simulink model "Test_DMP"  (R2018a)
settings: Solver=VariableStepAuto  StartTime=0.0  StopTime=2*tau  RelTol=1e-3
values from neighbouring files (symbols this model uses):
  Am = repmat(Am,1,6/length(Am))    [CostFCN.m]    (also in optimizeRobotMotion_openLoop.m; pFinal_runSim.m; simWalker_constraint.m)
  dt = .01    (= 0.01)    [Trajectory.m]    (also in rcp.m = 0.001)
  init_pos = Am'.*init_pos    [CostFCN.m]    (also in optimizeRobotMotion_openLoop.m; pFinal_runSim.m; simWalker_constraint.m)
  init_vel = Am'.*init_vel    [CostFCN.m]    (also in optimizeRobotMotion_openLoop.m; pFinal_runSim.m; simWalker_constraint.m)
  tau = params(1,2)    [CostFCN.m]    (also in Test_params.m = tau_nom; Trajectory.m = (2*pi)/omega; optimizeRobotMotion_openLoop.m = pFinal(1,2); pFinal_runSim.m = pFinal(1,2))
  Ym = Ym.*Am    [CostFCN.m]    (also in optimizeRobotMotion_openLoop.m; pFinal_runSim.m; simWalker_constraint.m)
undefined symbols (not defined in the file or in its folder): init_pos2, init_vel2, W, W2, Ym2
libraries: simulink_extras x6
(part 1 of 2)
settings Model: Creator=nozaripo  LastModifiedBy=nozaripo

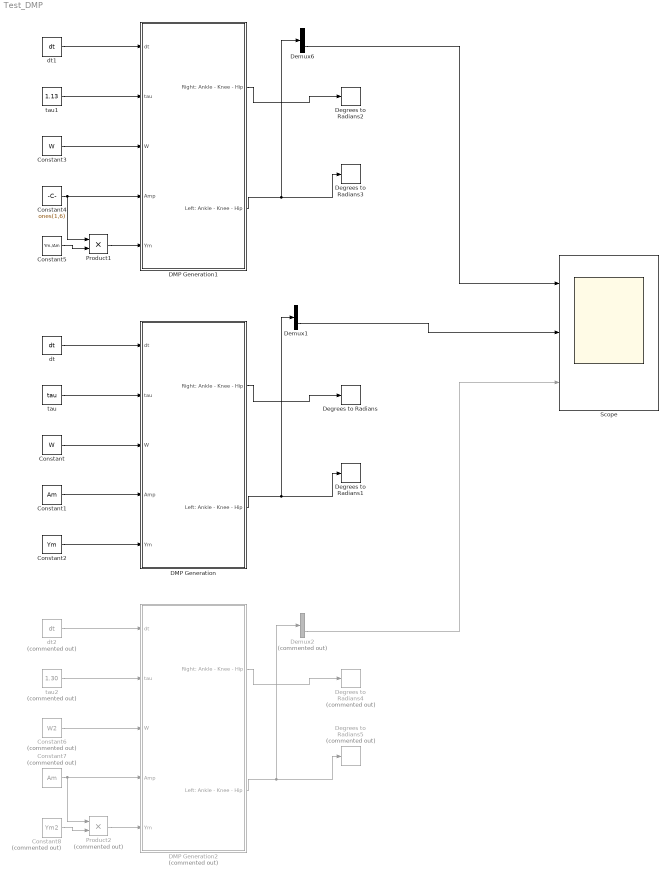
== system Test_DMP ==
  Constant : Constant  Value=W
  Constant1 : Constant  Value=Am
  Constant2 : Constant  Value=Ym
  Constant3 : Constant  Value=W
  Constant4 : Constant  Value=ones(1,6)
  Constant5 : Constant  Value=Ym./Am
  Constant6 : Constant  Commented=on  Value=W2
  Constant7 : Constant  Commented=on  Value=Am
  Constant8 : Constant  Commented=on  Value=Ym2
  DMP Generation : Subsystem
  DMP Generation1 : Subsystem
  DMP Generation2 : Subsystem  Commented=on
  Degrees to Radians{,1..3} (4 alike) : simulink_extras/Transformations/Degrees to Radians
  Degrees to Radians4 : simulink_extras/Transformations/Degrees to Radians  Commented=on
  Degrees to Radians5 : simulink_extras/Transformations/Degrees to Radians  Commented=on
  Demux1 : Demux  Outputs=3
  Demux2 : Demux  Commented=on  Outputs=3
  Demux6 : Demux  Outputs=3
  Product1 : Product
  Product2 : Product  Commented=on
  Scope : Scope  NumInputPorts=3
  dt : Constant  Value=dt
  dt1 : Constant  Value=dt
  dt2 : Constant  Commented=on  Value=dt
  tau : Constant  Value=tau
  tau1 : Constant  Value=1.13
  tau2 : Constant  Commented=on  Value=1.30
  wires:
  DMP Generation/2(Left: Ankle - Knee - Hip) -> Demux1/1, Degrees to Radians1/1
  DMP Generation/1(Right: Ankle - Knee - Hip) -> Degrees to Radians/1
  Constant/1 -> DMP Generation/3(W)
  Constant1/1 -> DMP Generation/4(Amp)
  Constant2/1 -> DMP Generation/5(Ym)
  tau/1 -> DMP Generation/2(tau)
  dt/1 -> DMP Generation/1(dt)
  dt1/1 -> DMP Generation1/1(dt)
  tau1/1 -> DMP Generation1/2(tau)
  Constant5/1 -> Product1/2
  Constant4/1 -> Product1/1, DMP Generation1/4(Amp)
  Constant3/1 -> DMP Generation1/3(W)
  DMP Generation1/1(Right: Ankle - Knee - Hip) -> Degrees to Radians2/1
  DMP Generation1/2(Left: Ankle - Knee - Hip) -> Demux6/1, Degrees to Radians3/1
  DMP Generation2/1(Right: Ankle - Knee - Hip) -> Degrees to Radians4/1
  DMP Generation2/2(Left: Ankle - Knee - Hip) -> Demux2/1, Degrees to Radians5/1
  Demux6/3 -> Scope/1
  Demux1/3 -> Scope/2
  Demux2/3 -> Scope/3
  Product1/1 -> DMP Generation1/5(Ym)
  Product2/1 -> DMP Generation2/5(Ym)
  Constant7/1 -> Product2/1, DMP Generation2/4(Amp)
  tau2/1 -> DMP Generation2/2(tau)
  Constant6/1 -> DMP Generation2/3(W)
  dt2/1 -> DMP Generation2/1(dt)
  Constant8/1 -> Product2/2

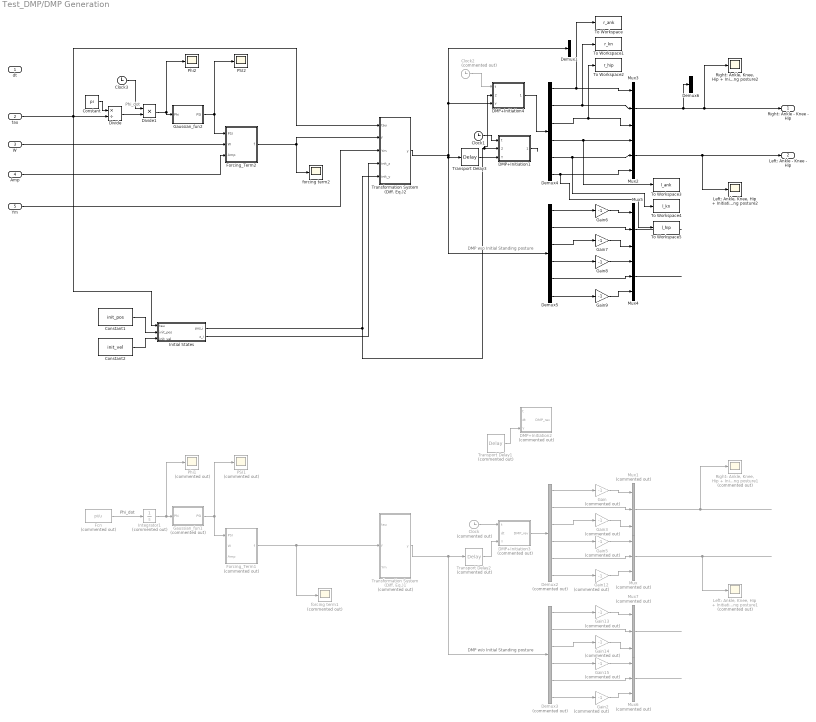
== system Test_DMP/DMP Generation ==
  note: Phi_dot
  note: DMP w/o Initial Standing posture
  note: Phi_dot
  note: DMP w/o Initial Standing posture
  dt : Inport
  tau : Inport  Port=2
  W : Inport  Port=3
  Amp : Inport  Port=4
  Ym : Inport  Port=5
  Clock : Clock  Commented=on
  Clock1 : Clock
  Clock2 : Clock  Commented=on
  Clock3 : Clock
  Constant : Constant  Value=pi
  Constant1 : Constant  Value=init_pos
  Constant2 : Constant  Value=init_vel
  DMP+Initiation1 : MATLAB Function  TreatAsAtomicUnit=on
  DMP+Initiation2 : MATLAB Function  Commented=on  TreatAsAtomicUnit=on
  DMP+Initiation3 : MATLAB Function  Commented=on  TreatAsAtomicUnit=on
  DMP+Initiation4 : MATLAB Function  TreatAsAtomicUnit=on
  Demux1 : Demux  Outputs=2
  Demux2 : Demux  Commented=on  Outputs=6
  Demux3 : Demux  Commented=on  Outputs=6
  Demux4 : Demux  Outputs=6
  Demux5 : Demux  Outputs=6
  Demux6 : Demux  Outputs=3
  Divide : Product  Inputs=*/
  Divide1 : Product  Inputs=**
  Fcn : Fcn  Commented=on  Expr=pi/u
  Forcing_Term1 : MATLAB Function  Commented=on  TreatAsAtomicUnit=on
  Forcing_Term2 : MATLAB Function  TreatAsAtomicUnit=on
  Gain{,2..3,5,12..15} (8 alike) : Gain  Commented=on  Gain=-1
  Gain{6..9} (4 alike) : Gain  Gain=-1
  Gaussian_fun1 : MATLAB Function  Commented=on  TreatAsAtomicUnit=on
  Gaussian_fun2 : MATLAB Function  TreatAsAtomicUnit=on
  Initial States : MATLAB Function  TreatAsAtomicUnit=on
  Integrator1 : Integrator  Commented=on
  "Left: Ankle, Knee, Hip + Initiatial standing posture1" : Scope  Commented=on
  "Left: Ankle, Knee, Hip + Initiatial standing posture2" : Scope
  Mux{,1,6..7} (4 alike) : Mux  Commented=on  Inputs=3
  Mux{2..5} (4 alike) : Mux  Inputs=3
  PSI1 : Scope  Commented=on
  PSI2 : Scope
  Phi1 : Scope  Commented=on
  Phi2 : Scope
  "Right: Ankle, Knee, Hip + Initiatial standing posture1" : Scope  Commented=on
  "Right: Ankle, Knee, Hip + Initiatial standing posture2" : Scope
  To Workspace : ToWorkspace  VariableName=r_ank  SampleTime=-1
      settings: Save2DSignal=2-D array (concatenate along first dimension)
  To Workspace1 : ToWorkspace  VariableName=r_kn  SampleTime=-1
      settings: Save2DSignal=2-D array (concatenate along first dimension)
  To Workspace2 : ToWorkspace  VariableName=r_hip  SampleTime=-1
      settings: Save2DSignal=2-D array (concatenate along first dimension)
  To Workspace3 : ToWorkspace  VariableName=l_ank  SampleTime=-1
      settings: Save2DSignal=2-D array (concatenate along first dimension)
  To Workspace4 : ToWorkspace  VariableName=l_kn  SampleTime=-1
      settings: Save2DSignal=2-D array (concatenate along first dimension)
  To Workspace5 : ToWorkspace  VariableName=l_hip  SampleTime=-1
      settings: Save2DSignal=2-D array (concatenate along first dimension)
  Transformation System (Diff. Eq.)1 : Subsystem  Commented=on
  Transformation System (Diff. Eq.)2 : Subsystem
  Transport Delay1 : TransportDelay  Commented=on  DelayTime=.45
  Transport Delay2 : TransportDelay  Commented=on  DelayTime=.55
  Transport Delay3 : TransportDelay  DelayTime=.67
  forcing term1 : Scope  Commented=on
  forcing term2 : Scope
  Right: Ankle - Knee - Hip : Outport
  Left: Ankle - Knee - Hip : Outport  Port=2
  wires:
  Demux2/3 -> Gain3/1
  Gain14/1 -> Mux7/3
  Demux2/5 -> Mux/2
  Demux2/6 -> Gain12/1
  Mux1/1 -> "Right: Ankle, Knee, Hip + Initiatial standing posture1"/1
  Demux3/5 -> Mux6/2
  Demux3/2 -> Mux7/2
  Gain3/1 -> Mux1/3
  Gain15/1 -> Mux6/1
  Demux2/4 -> Gain5/1
  Demux3/3 -> Gain14/1
  Mux6/1 -> ?
  Gaussian_fun1/1(PSI) -> PSI1/1, Forcing_Term1/1(PSI)
  Mux7/1 -> ?
  DMP+Initiation3/1(DMP_rev) -> Demux2/1
  Gain2/1 -> Mux6/3
  Transformation System (Diff. Eq.)1/1(y) -> Transport Delay2/1, Demux3/1
  Forcing_Term1/1(f) -> forcing term1/1, Transformation System (Diff. Eq.)1/2(f)
  Gain/1 -> Mux1/1
  Demux3/4 -> Gain15/1
  Mux/1 -> "Left: Ankle, Knee, Hip + Initiatial standing posture1"/1
  Fcn/1 -> Integrator1/1
  Demux2/2 -> Mux1/2
  Integrator1/1 -> Phi1/1, Gaussian_fun1/1(Phi)
  Gain5/1 -> Mux/1
  Demux3/1 -> Gain13/1
  Demux3/6 -> Gain2/1
  Demux2/1 -> Gain/1
  ? -> Forcing_Term1/3(Amp)
  ? -> Transformation System (Diff. Eq.)1/3(Ym)
  Gain12/1 -> Mux/3
  ? -> Fcn/1, Transformation System (Diff. Eq.)1/1(tau)
  ? -> Forcing_Term1/2(W)
  Gain13/1 -> Mux7/1
  ? -> DMP+Initiation2/1(t)
  Transport Delay1/1 -> DMP+Initiation2/3(Y)
  ? -> DMP+Initiation3/2(dt)
  Clock/1 -> DMP+Initiation3/1(t)
  Transport Delay2/1 -> DMP+Initiation3/3(Y)
  DMP+Initiation1/1(DMP_rev) -> ?
  Divide/1 -> Divide1/2
  Mux5/1 -> ?
  Forcing_Term2/1(f) -> Transformation System (Diff. Eq.)2/2(f), forcing term2/1
  Demux4/6 -> Mux2/3, To Workspace5/1
  Ym/1 -> Transformation System (Diff. Eq.)2/3(Ym)
  Demux5/1 -> Gain6/1
  Demux5/2 -> Mux5/2
  Mux2/1 -> Left: Ankle - Knee - Hip/1, "Left: Ankle, Knee, Hip + Initiatial standing posture2"/1
  Demux5/4 -> Gain8/1
  Transport Delay3/1 -> DMP+Initiation1/3(Y)
  Constant/1 -> Divide/1
  Demux4/5 -> To Workspace4/1, Mux2/2
  Gain9/1 -> Mux4/3
  Clock1/1 -> DMP+Initiation1/1(t)
  Gain8/1 -> Mux4/1
  Demux4/3 -> Mux3/3, To Workspace2/1
  Gain7/1 -> Mux5/3
  Demux5/3 -> Gain7/1
  Demux5/6 -> Gain9/1
  Amp/1 -> Forcing_Term2/3(Amp)
  Demux5/5 -> Mux4/2
  Gaussian_fun2/1(PSI) -> PSI2/1, Forcing_Term2/1(PSI)
  W/1 -> Forcing_Term2/2(W)
  Demux4/4 -> Mux2/1, To Workspace3/1
  Demux4/1 -> Mux3/1, To Workspace/1
  Mux4/1 -> ?
  Transformation System (Diff. Eq.)2/1(y) -> Transport Delay3/1, Demux5/1, DMP+Initiation4/3(Y), Demux1/1
  Demux4/2 -> To Workspace1/1, Mux3/2
  Mux3/1 -> Demux6/1, Right: Ankle - Knee - Hip/1, "Right: Ankle, Knee, Hip + Initiatial standing posture2"/1
  Divide1/1 -> Gaussian_fun2/1(Phi), Phi2/1
  Gain6/1 -> Mux5/1
  Constant2/1 -> Initial States/3(init_vel)
  Constant1/1 -> Initial States/2(init_pos)
  Initial States/2(z_i) -> Transformation System (Diff. Eq.)2/4(init_z)
  Initial States/1(pos_i) -> Transformation System (Diff. Eq.)2/5(init_y), DMP+Initiation4/2(init_pos), DMP+Initiation1/2(init_pos)
  tau/1 -> Transformation System (Diff. Eq.)2/1(tau), Initial States/1(tau), Divide/2
  Clock2/1 -> DMP+Initiation4/1(t)
  DMP+Initiation4/1(DMP_rev) -> Demux4/1
  Clock3/1 -> Divide1/1

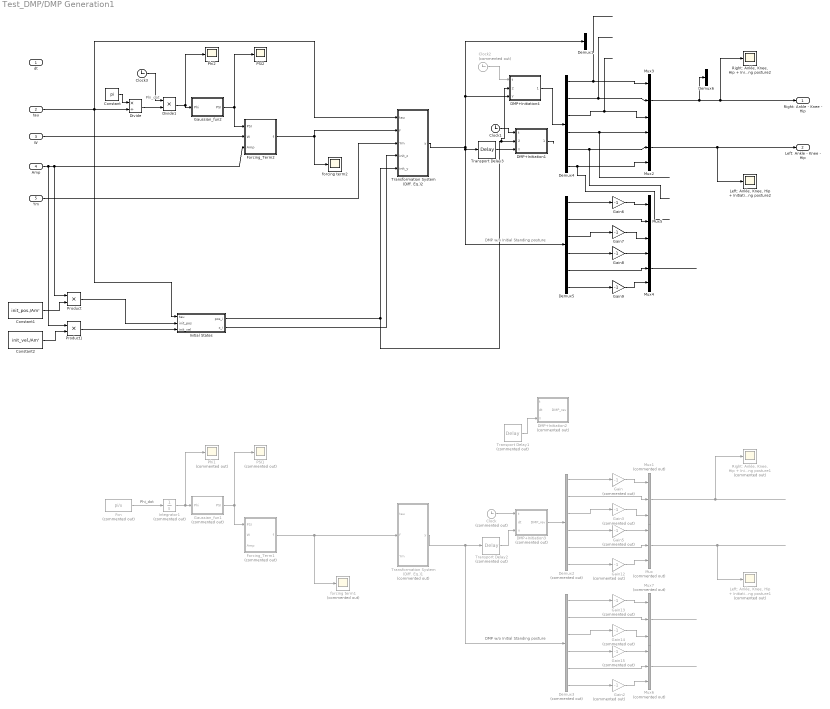
== system Test_DMP/DMP Generation1 ==
  note: DMP w/o Initial Standing posture
  note: Phi_dot
  note: DMP w/o Initial Standing posture
  note: Phi_dot
  dt : Inport
  tau : Inport  Port=2
  W : Inport  Port=3
  Amp : Inport  Port=4
  Ym : Inport  Port=5
  Clock : Clock  Commented=on
  Clock1 : Clock
  Clock2 : Clock  Commented=on
  Clock3 : Clock
  Constant : Constant  Value=pi
  Constant1 : Constant  Value=init_pos./Am'
  Constant2 : Constant  Value=init_vel./Am'
  DMP+Initiation1 : MATLAB Function  TreatAsAtomicUnit=on
  DMP+Initiation2 : MATLAB Function  Commented=on  TreatAsAtomicUnit=on
  DMP+Initiation3 : MATLAB Function  Commented=on  TreatAsAtomicUnit=on
  DMP+Initiation4 : MATLAB Function  TreatAsAtomicUnit=on
  Demux1 : Demux  Outputs=2
  Demux2 : Demux  Commented=on  Outputs=6
  Demux3 : Demux  Commented=on  Outputs=6
  Demux4 : Demux  Outputs=6
  Demux5 : Demux  Outputs=6
  Demux6 : Demux  Outputs=3
  Divide : Product  Inputs=*/
  Divide1 : Product  Inputs=**
  Fcn : Fcn  Commented=on  Expr=pi/u
  Forcing_Term1 : MATLAB Function  Commented=on  TreatAsAtomicUnit=on
  Forcing_Term2 : MATLAB Function  TreatAsAtomicUnit=on
  Gain{,2..3,5,12..15} (8 alike) : Gain  Commented=on  Gain=-1
  Gain{6..9} (4 alike) : Gain  Gain=-1
  Gaussian_fun1 : MATLAB Function  Commented=on  TreatAsAtomicUnit=on
  Gaussian_fun2 : MATLAB Function  TreatAsAtomicUnit=on
  Initial States : MATLAB Function  TreatAsAtomicUnit=on
  Integrator1 : Integrator  Commented=on
  "Left: Ankle, Knee, Hip + Initiatial standing posture1" : Scope  Commented=on
  "Left: Ankle, Knee, Hip + Initiatial standing posture2" : Scope
  Mux{,1,6..7} (4 alike) : Mux  Commented=on  Inputs=3
  Mux{2..5} (4 alike) : Mux  Inputs=3
  PSI1 : Scope  Commented=on
  PSI2 : Scope
  Phi1 : Scope  Commented=on
  Phi2 : Scope
  Product : Product
  Product1 : Product
  "Right: Ankle, Knee, Hip + Initiatial standing posture1" : Scope  Commented=on
  "Right: Ankle, Knee, Hip + Initiatial standing posture2" : Scope
  Transformation System (Diff. Eq.)1 : Subsystem  Commented=on
  Transformation System (Diff. Eq.)2 : Subsystem
  Transport Delay1 : TransportDelay  Commented=on  DelayTime=.45
  Transport Delay2 : TransportDelay  Commented=on  DelayTime=.55
  Transport Delay3 : TransportDelay  DelayTime=.67
  forcing term1 : Scope  Commented=on
  forcing term2 : Scope
  Right: Ankle - Knee - Hip : Outport
  Left: Ankle - Knee - Hip : Outport  Port=2
  wires:
  Clock3/1 -> Divide1/1
  DMP+Initiation4/1(DMP_rev) -> Demux4/1
  Clock2/1 -> DMP+Initiation4/1(t)
  tau/1 -> Divide/2, Initial States/1(tau), Transformation System (Diff. Eq.)2/1(tau)
  Initial States/1(pos_i) -> DMP+Initiation1/2(init_pos), DMP+Initiation4/2(init_pos), Transformation System (Diff. Eq.)2/5(init_y)
  Initial States/2(z_i) -> Transformation System (Diff. Eq.)2/4(init_z)
  Constant1/1 -> Product/2
  Gain6/1 -> Mux5/1
  Divide1/1 -> Phi2/1, Gaussian_fun2/1(Phi)
  Mux3/1 -> "Right: Ankle, Knee, Hip + Initiatial standing posture2"/1, Right: Ankle - Knee - Hip/1, Demux6/1
  Demux4/2 -> Mux3/2
  Transformation System (Diff. Eq.)2/1(y) -> Demux1/1, DMP+Initiation4/3(Y), Demux5/1, Transport Delay3/1
  Mux4/1 -> ?
  Demux4/1 -> Mux3/1
  Demux4/4 -> Mux2/1
  W/1 -> Forcing_Term2/2(W)
  Gaussian_fun2/1(PSI) -> Forcing_Term2/1(PSI), PSI2/1
  Demux5/5 -> Mux4/2
  Amp/1 -> Product1/1, Product/1, Forcing_Term2/3(Amp)
  Demux5/6 -> Gain9/1
  Demux5/3 -> Gain7/1
  Gain7/1 -> Mux5/3
  Demux4/3 -> Mux3/3
  Gain8/1 -> Mux4/1
  Clock1/1 -> DMP+Initiation1/1(t)
  Gain9/1 -> Mux4/3
  Demux4/5 -> Mux2/2
  Constant/1 -> Divide/1
  Transport Delay3/1 -> DMP+Initiation1/3(Y)
  Demux5/4 -> Gain8/1
  Mux2/1 -> "Left: Ankle, Knee, Hip + Initiatial standing posture2"/1, Left: Ankle - Knee - Hip/1
  Demux5/2 -> Mux5/2
  Demux5/1 -> Gain6/1
  Ym/1 -> Transformation System (Diff. Eq.)2/3(Ym)
  Demux4/6 -> Mux2/3
  Forcing_Term2/1(f) -> forcing term2/1, Transformation System (Diff. Eq.)2/2(f)
  Divide/1 -> Divide1/2
  DMP+Initiation1/1(DMP_rev) -> ?
  Transport Delay2/1 -> DMP+Initiation3/3(Y)
  Clock/1 -> DMP+Initiation3/1(t)
  ? -> DMP+Initiation3/2(dt)
  Transport Delay1/1 -> DMP+Initiation2/3(Y)
  ? -> DMP+Initiation2/1(t)
  Gain13/1 -> Mux7/1
  ? -> Forcing_Term1/2(W)
  ? -> Transformation System (Diff. Eq.)1/1(tau), Fcn/1
  Gain12/1 -> Mux/3
  ? -> Transformation System (Diff. Eq.)1/3(Ym)
  ? -> Forcing_Term1/3(Amp)
  Demux2/1 -> Gain/1
  Demux3/6 -> Gain2/1
  Demux3/1 -> Gain13/1
  Gain5/1 -> Mux/1
  Integrator1/1 -> Gaussian_fun1/1(Phi), Phi1/1
  Demux2/2 -> Mux1/2
  Fcn/1 -> Integrator1/1
  Mux/1 -> "Left: Ankle, Knee, Hip + Initiatial standing posture1"/1
  Demux3/4 -> Gain15/1
  Gain/1 -> Mux1/1
  Forcing_Term1/1(f) -> Transformation System (Diff. Eq.)1/2(f), forcing term1/1
  Transformation System (Diff. Eq.)1/1(y) -> Demux3/1, Transport Delay2/1
  Gain2/1 -> Mux6/3
  DMP+Initiation3/1(DMP_rev) -> Demux2/1
  Mux7/1 -> ?
  Gaussian_fun1/1(PSI) -> Forcing_Term1/1(PSI), PSI1/1
  Mux6/1 -> ?
  Demux3/3 -> Gain14/1
  Demux2/4 -> Gain5/1
  Gain15/1 -> Mux6/1
  Gain3/1 -> Mux1/3
  Demux3/2 -> Mux7/2
  Demux3/5 -> Mux6/2
  Mux1/1 -> "Right: Ankle, Knee, Hip + Initiatial standing posture1"/1
  Demux2/6 -> Gain12/1
  Demux2/5 -> Mux/2
  Gain14/1 -> Mux7/3
  Demux2/3 -> Gain3/1
  Product/1 -> Initial States/2(init_pos)
  Constant2/1 -> Product1/2
  Product1/1 -> Initial States/3(init_vel)

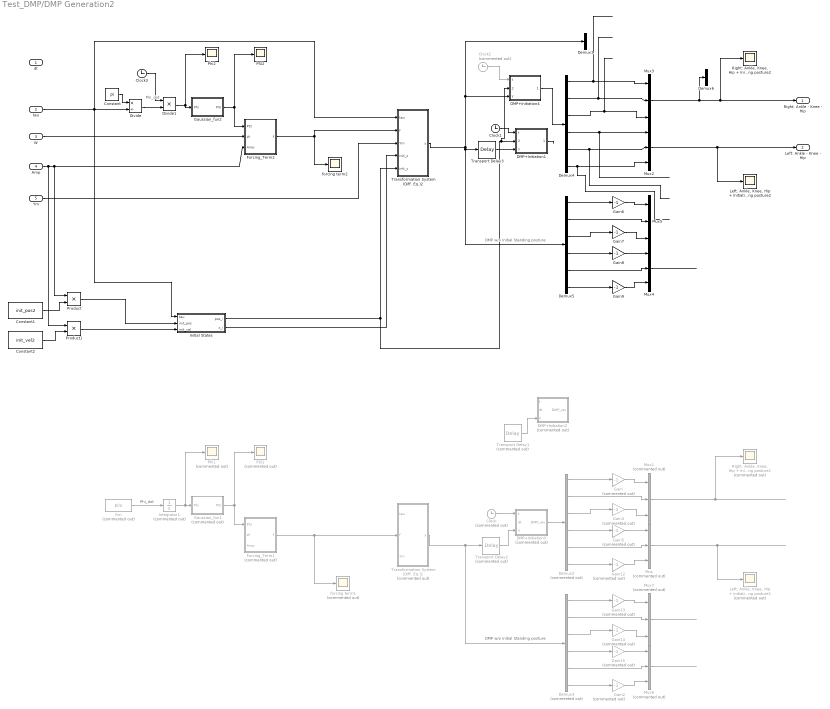
== system Test_DMP/DMP Generation2 ==
  note: DMP w/o Initial Standing posture
  note: Phi_dot
  note: DMP w/o Initial Standing posture
  note: Phi_dot
  dt : Inport
  tau : Inport  Port=2
  W : Inport  Port=3
  Amp : Inport  Port=4
  Ym : Inport  Port=5
  Clock : Clock  Commented=on
  Clock1 : Clock
  Clock2 : Clock  Commented=on
  Clock3 : Clock
  Constant : Constant  Value=pi
  Constant1 : Constant  Value=init_pos2
  Constant2 : Constant  Value=init_vel2
  DMP+Initiation1 : MATLAB Function  TreatAsAtomicUnit=on
  DMP+Initiation2 : MATLAB Function  Commented=on  TreatAsAtomicUnit=on
  DMP+Initiation3 : MATLAB Function  Commented=on  TreatAsAtomicUnit=on
  DMP+Initiation4 : MATLAB Function  TreatAsAtomicUnit=on
  Demux1 : Demux  Outputs=2
  Demux2 : Demux  Commented=on  Outputs=6
  Demux3 : Demux  Commented=on  Outputs=6
  Demux4 : Demux  Outputs=6
  Demux5 : Demux  Outputs=6
  Demux6 : Demux  Outputs=3
  Divide : Product  Inputs=*/
  Divide1 : Product  Inputs=**
  Fcn : Fcn  Commented=on  Expr=pi/u
  Forcing_Term1 : MATLAB Function  Commented=on  TreatAsAtomicUnit=on
  Forcing_Term2 : MATLAB Function  TreatAsAtomicUnit=on
  Gain{,2..3,5,12..15} (8 alike) : Gain  Commented=on  Gain=-1
  Gain{6..9} (4 alike) : Gain  Gain=-1
  Gaussian_fun1 : MATLAB Function  Commented=on  TreatAsAtomicUnit=on
  Gaussian_fun2 : MATLAB Function  TreatAsAtomicUnit=on
  Initial States : MATLAB Function  TreatAsAtomicUnit=on
  Integrator1 : Integrator  Commented=on
  "Left: Ankle, Knee, Hip + Initiatial standing posture1" : Scope  Commented=on
  "Left: Ankle, Knee, Hip + Initiatial standing posture2" : Scope
  Mux{,1,6..7} (4 alike) : Mux  Commented=on  Inputs=3
  Mux{2..5} (4 alike) : Mux  Inputs=3
  PSI1 : Scope  Commented=on
  PSI2 : Scope
  Phi1 : Scope  Commented=on
  Phi2 : Scope
  Product : Product
  Product1 : Product
  "Right: Ankle, Knee, Hip + Initiatial standing posture1" : Scope  Commented=on
  "Right: Ankle, Knee, Hip + Initiatial standing posture2" : Scope
  Transformation System (Diff. Eq.)1 : Subsystem  Commented=on
  Transformation System (Diff. Eq.)2 : Subsystem
  Transport Delay1 : TransportDelay  Commented=on  DelayTime=.45
  Transport Delay2 : TransportDelay  Commented=on  DelayTime=.55
  Transport Delay3 : TransportDelay  DelayTime=.67
  forcing term1 : Scope  Commented=on
  forcing term2 : Scope
  Right: Ankle - Knee - Hip : Outport
  Left: Ankle - Knee - Hip : Outport  Port=2
  wires:
  Clock3/1 -> Divide1/1
  DMP+Initiation4/1(DMP_rev) -> Demux4/1
  Clock2/1 -> DMP+Initiation4/1(t)
  tau/1 -> Divide/2, Initial States/1(tau), Transformation System (Diff. Eq.)2/1(tau)
  Initial States/1(pos_i) -> DMP+Initiation1/2(init_pos), DMP+Initiation4/2(init_pos), Transformation System (Diff. Eq.)2/5(init_y)
  Initial States/2(z_i) -> Transformation System (Diff. Eq.)2/4(init_z)
  Constant1/1 -> Product/2
  Gain6/1 -> Mux5/1
  Divide1/1 -> Phi2/1, Gaussian_fun2/1(Phi)
  Mux3/1 -> "Right: Ankle, Knee, Hip + Initiatial standing posture2"/1, Right: Ankle - Knee - Hip/1, Demux6/1
  Demux4/2 -> Mux3/2
  Transformation System (Diff. Eq.)2/1(y) -> Demux1/1, DMP+Initiation4/3(Y), Demux5/1, Transport Delay3/1
  Mux4/1 -> ?
  Demux4/1 -> Mux3/1
  Demux4/4 -> Mux2/1
  W/1 -> Forcing_Term2/2(W)
  Gaussian_fun2/1(PSI) -> Forcing_Term2/1(PSI), PSI2/1
  Demux5/5 -> Mux4/2
  Amp/1 -> Product1/1, Product/1, Forcing_Term2/3(Amp)
  Demux5/6 -> Gain9/1
  Demux5/3 -> Gain7/1
  Gain7/1 -> Mux5/3
  Demux4/3 -> Mux3/3
  Gain8/1 -> Mux4/1
  Clock1/1 -> DMP+Initiation1/1(t)
  Gain9/1 -> Mux4/3
  Demux4/5 -> Mux2/2
  Constant/1 -> Divide/1
  Transport Delay3/1 -> DMP+Initiation1/3(Y)
  Demux5/4 -> Gain8/1
  Mux2/1 -> "Left: Ankle, Knee, Hip + Initiatial standing posture2"/1, Left: Ankle - Knee - Hip/1
  Demux5/2 -> Mux5/2
  Demux5/1 -> Gain6/1
  Ym/1 -> Transformation System (Diff. Eq.)2/3(Ym)
  Demux4/6 -> Mux2/3
  Forcing_Term2/1(f) -> forcing term2/1, Transformation System (Diff. Eq.)2/2(f)
  Divide/1 -> Divide1/2
  DMP+Initiation1/1(DMP_rev) -> ?
  Transport Delay2/1 -> DMP+Initiation3/3(Y)
  Clock/1 -> DMP+Initiation3/1(t)
  ? -> DMP+Initiation3/2(dt)
  Transport Delay1/1 -> DMP+Initiation2/3(Y)
  ? -> DMP+Initiation2/1(t)
  Gain13/1 -> Mux7/1
  ? -> Forcing_Term1/2(W)
  ? -> Transformation System (Diff. Eq.)1/1(tau), Fcn/1
  Gain12/1 -> Mux/3
  ? -> Transformation System (Diff. Eq.)1/3(Ym)
  ? -> Forcing_Term1/3(Amp)
  Demux2/1 -> Gain/1
  Demux3/6 -> Gain2/1
  Demux3/1 -> Gain13/1
  Gain5/1 -> Mux/1
  Integrator1/1 -> Gaussian_fun1/1(Phi), Phi1/1
  Demux2/2 -> Mux1/2
  Fcn/1 -> Integrator1/1
  Mux/1 -> "Left: Ankle, Knee, Hip + Initiatial standing posture1"/1
  Demux3/4 -> Gain15/1
  Gain/1 -> Mux1/1
  Forcing_Term1/1(f) -> Transformation System (Diff. Eq.)1/2(f), forcing term1/1
  Transformation System (Diff. Eq.)1/1(y) -> Demux3/1, Transport Delay2/1
  Gain2/1 -> Mux6/3
  DMP+Initiation3/1(DMP_rev) -> Demux2/1
  Mux7/1 -> ?
  Gaussian_fun1/1(PSI) -> Forcing_Term1/1(PSI), PSI1/1
  Mux6/1 -> ?
  Demux3/3 -> Gain14/1
  Demux2/4 -> Gain5/1
  Gain15/1 -> Mux6/1
  Gain3/1 -> Mux1/3
  Demux3/2 -> Mux7/2
  Demux3/5 -> Mux6/2
  Mux1/1 -> "Right: Ankle, Knee, Hip + Initiatial standing posture1"/1
  Demux2/6 -> Gain12/1
  Demux2/5 -> Mux/2
  Gain14/1 -> Mux7/3
  Demux2/3 -> Gain3/1
  Product/1 -> Initial States/2(init_pos)
  Constant2/1 -> Product1/2
  Product1/1 -> Initial States/3(init_vel)

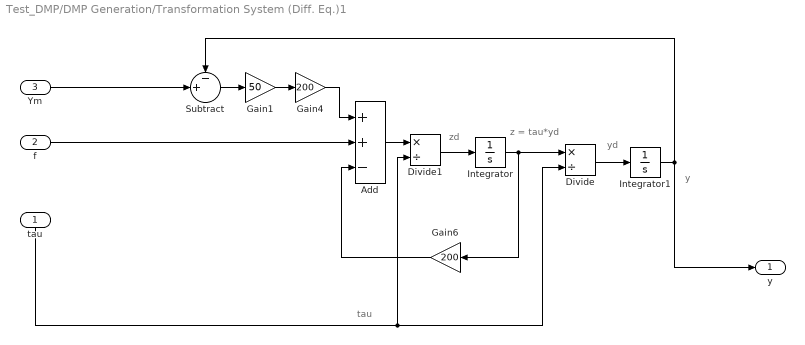
== system Test_DMP/DMP Generation/Transformation System (Diff. Eq.)1 ==
  note: y
  note: zd
  note: tau
  note: yd
  note: z = tau*yd
  tau : Inport
  f : Inport  Port=2
  Ym : Inport  Port=3
  Add : Sum  Inputs=++-
  Divide : Product  Inputs=*/
  Divide1 : Product  Inputs=*/
  Gain1 : Gain  Gain=50
  Gain4 : Gain  Gain=200
  Gain6 : Gain  Gain=200
  Integrator : Integrator
  Integrator1 : Integrator
  Subtract : Sum  Inputs=-+|
  y : Outport
  wires:
  Divide/1 -> Integrator1/1
  Add/1 -> Divide1/1
  Gain1/1 -> Gain4/1
  Gain4/1 -> Add/1
  Subtract/1 -> Gain1/1
  Divide1/1 -> Integrator/1
  tau/1 -> Divide/2, Divide1/2
  f/1 -> Add/2
  Integrator1/1 -> y/1, Subtract/1
  Integrator/1 -> Gain6/1, Divide/1
  Gain6/1 -> Add/3
  Ym/1 -> Subtract/2

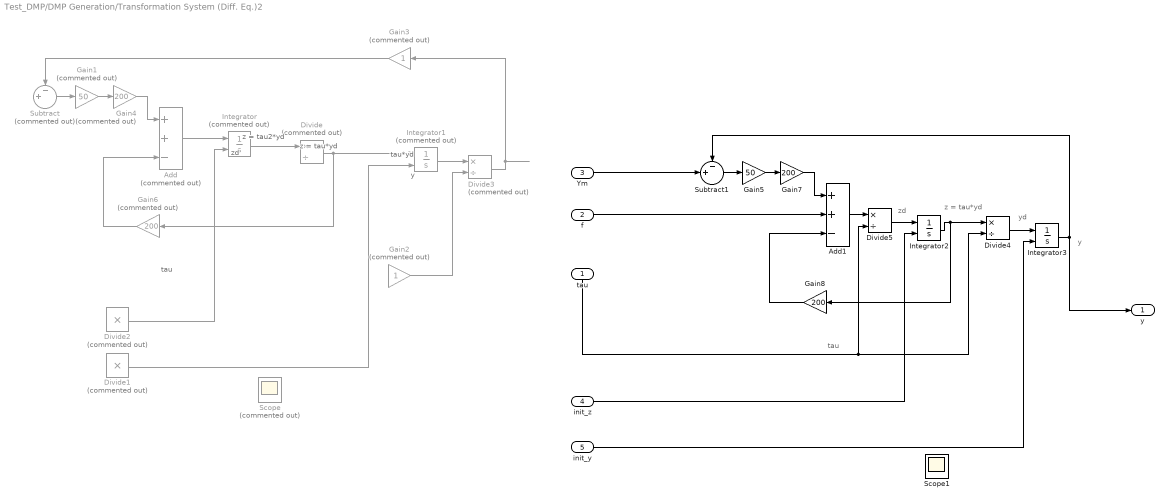
== system Test_DMP/DMP Generation/Transformation System (Diff. Eq.)2 ==
  note: y
  note: zd
  note: tau
  note: tau*yd
  note: z = tau2*yd
  note: z = tau*yd
  note: y
  note: zd
  note: tau
  note: yd
  note: z = tau*yd
  tau : Inport
  f : Inport  Port=2
  Ym : Inport  Port=3
  init_z : Inport  Port=4
  init_y : Inport  Port=5
  Add : Sum  Commented=on  Inputs=++-
  Add1 : Sum  Inputs=++-
  Divide : Product  Commented=on  Inputs=*/
  Divide1 : Product  Commented=on  Inputs=**
  Divide2 : Product  Commented=on  Inputs=**
  Divide3 : Product  Commented=on  Inputs=*/
  Divide4 : Product  Inputs=*/
  Divide5 : Product  Inputs=*/
  Gain1 : Gain  Commented=on  Gain=50
  Gain2 : Gain  Commented=on
  Gain3 : Gain  Commented=on
  Gain4 : Gain  Commented=on  Gain=200
  Gain5 : Gain  Gain=50
  Gain6 : Gain  Commented=on  Gain=200
  Gain7 : Gain  Gain=200
  Gain8 : Gain  Gain=200
  Integrator : Integrator  Commented=on  InitialConditionSource=external  LimitOutput=on
  Integrator1 : Integrator  Commented=on  InitialConditionSource=external
  Integrator2 : Integrator  InitialConditionSource=external
  Integrator3 : Integrator  InitialConditionSource=external
  Scope : Scope  Commented=on
  Scope1 : Scope
  Subtract : Sum  Commented=on  Inputs=-+|
  Subtract1 : Sum  Inputs=-+|
  y : Outport
  wires:
  Divide/1 -> Gain6/1, Integrator1/1
  Gain1/1 -> Gain4/1
  Gain4/1 -> Add/1
  Subtract/1 -> Gain1/1
  Add/1 -> Integrator/1
  ? -> Divide1/1, Divide2/1, Gain2/1, Divide/2
  ? -> Add/2
  Divide3/1 -> Gain3/1
  Integrator/1 -> Divide/1
  Gain6/1 -> Add/3
  ? -> Subtract/2
  ? -> Divide2/2
  ? -> Divide1/2
  Divide2/1 -> Integrator/2
  Divide1/1 -> Integrator1/2
  Integrator1/1 -> Divide3/1
  Gain2/1 -> Divide3/2
  Gain3/1 -> Subtract/1
  init_y/1 -> Integrator3/2
  Ym/1 -> Subtract1/2
  Integrator2/1 -> Gain8/1, Divide4/1
  init_z/1 -> Integrator2/2
  Gain8/1 -> Add1/3
  Integrator3/1 -> Subtract1/1, y/1
  f/1 -> Add1/2
  Divide5/1 -> Integrator2/1
  Gain7/1 -> Add1/1
  tau/1 -> Divide4/2, Divide5/2
  Subtract1/1 -> Gain5/1
  Gain5/1 -> Gain7/1
  Add1/1 -> Divide5/1
  Divide4/1 -> Integrator3/1

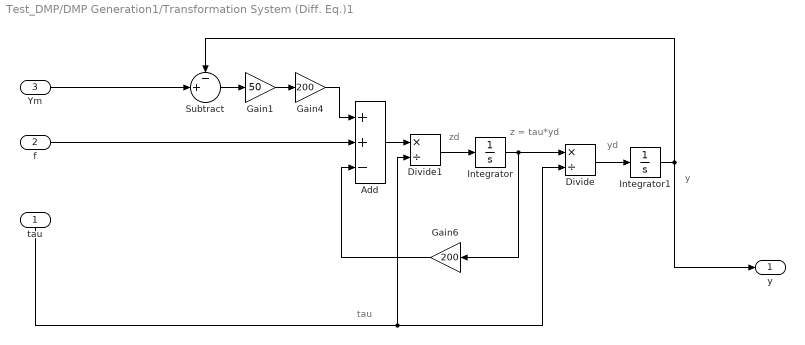
== system Test_DMP/DMP Generation1/Transformation System (Diff. Eq.)1 ==
  note: z = tau*yd
  note: yd
  note: tau
  note: zd
  note: y
  tau : Inport
  f : Inport  Port=2
  Ym : Inport  Port=3
  Add : Sum  Inputs=++-
  Divide : Product  Inputs=*/
  Divide1 : Product  Inputs=*/
  Gain1 : Gain  Gain=50
  Gain4 : Gain  Gain=200
  Gain6 : Gain  Gain=200
  Integrator : Integrator
  Integrator1 : Integrator
  Subtract : Sum  Inputs=-+|
  y : Outport
  wires:
  Ym/1 -> Subtract/2
  Gain6/1 -> Add/3
  Integrator/1 -> Divide/1, Gain6/1
  Integrator1/1 -> Subtract/1, y/1
  f/1 -> Add/2
  tau/1 -> Divide1/2, Divide/2
  Divide1/1 -> Integrator/1
  Subtract/1 -> Gain1/1
  Gain4/1 -> Add/1
  Gain1/1 -> Gain4/1
  Add/1 -> Divide1/1
  Divide/1 -> Integrator1/1

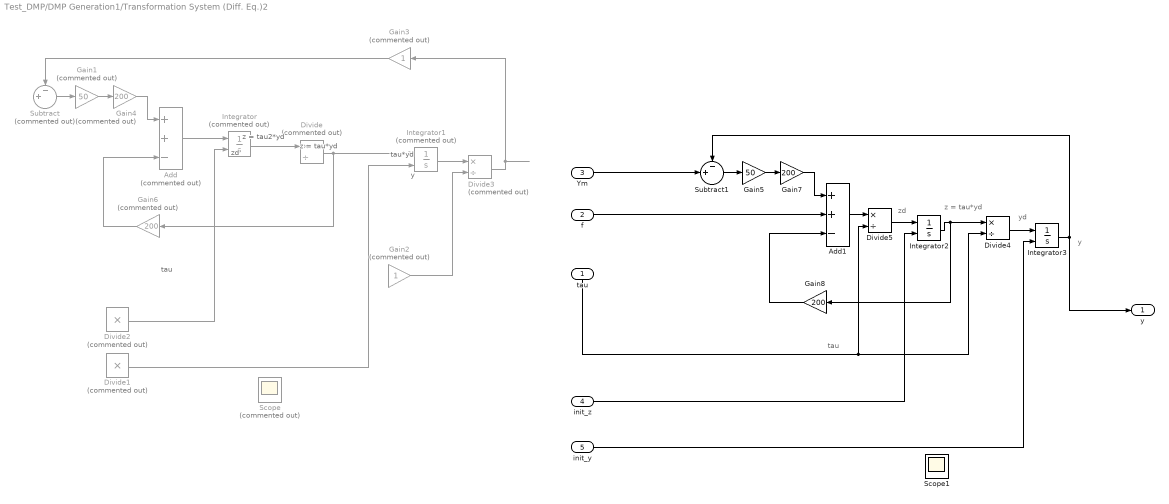
== system Test_DMP/DMP Generation1/Transformation System (Diff. Eq.)2 ==
  note: z = tau*yd
  note: yd
  note: tau
  note: zd
  note: y
  note: z = tau*yd
  note: z = tau2*yd
  note: tau*yd
  note: tau
  note: zd
  note: y
  tau : Inport
  f : Inport  Port=2
  Ym : Inport  Port=3
  init_z : Inport  Port=4
  init_y : Inport  Port=5
  Add : Sum  Commented=on  Inputs=++-
  Add1 : Sum  Inputs=++-
  Divide : Product  Commented=on  Inputs=*/
  Divide1 : Product  Commented=on  Inputs=**
  Divide2 : Product  Commented=on  Inputs=**
  Divide3 : Product  Commented=on  Inputs=*/
  Divide4 : Product  Inputs=*/
  Divide5 : Product  Inputs=*/
  Gain1 : Gain  Commented=on  Gain=50
  Gain2 : Gain  Commented=on
  Gain3 : Gain  Commented=on
  Gain4 : Gain  Commented=on  Gain=200
  Gain5 : Gain  Gain=50
  Gain6 : Gain  Commented=on  Gain=200
  Gain7 : Gain  Gain=200
  Gain8 : Gain  Gain=200
  Integrator : Integrator  Commented=on  InitialConditionSource=external  LimitOutput=on
  Integrator1 : Integrator  Commented=on  InitialConditionSource=external
  Integrator2 : Integrator  InitialConditionSource=external
  Integrator3 : Integrator  InitialConditionSource=external
  Scope : Scope  Commented=on
  Scope1 : Scope
  Subtract : Sum  Commented=on  Inputs=-+|
  Subtract1 : Sum  Inputs=-+|
  y : Outport
  wires:
  Divide4/1 -> Integrator3/1
  Add1/1 -> Divide5/1
  Gain5/1 -> Gain7/1
  Subtract1/1 -> Gain5/1
  tau/1 -> Divide5/2, Divide4/2
  Gain7/1 -> Add1/1
  Divide5/1 -> Integrator2/1
  f/1 -> Add1/2
  Integrator3/1 -> y/1, Subtract1/1
  Gain8/1 -> Add1/3
  init_z/1 -> Integrator2/2
  Integrator2/1 -> Divide4/1, Gain8/1
  Ym/1 -> Subtract1/2
  init_y/1 -> Integrator3/2
  Gain3/1 -> Subtract/1
  Gain2/1 -> Divide3/2
  Integrator1/1 -> Divide3/1
  Divide1/1 -> Integrator1/2
  Divide2/1 -> Integrator/2
  ? -> Divide1/2
  ? -> Divide2/2
  ? -> Subtract/2
  Gain6/1 -> Add/3
  Integrator/1 -> Divide/1
  Divide3/1 -> Gain3/1
  ? -> Add/2
  ? -> Divide/2, Gain2/1, Divide2/1, Divide1/1
  Add/1 -> Integrator/1
  Subtract/1 -> Gain1/1
  Gain4/1 -> Add/1
  Gain1/1 -> Gain4/1
  Divide/1 -> Integrator1/1, Gain6/1

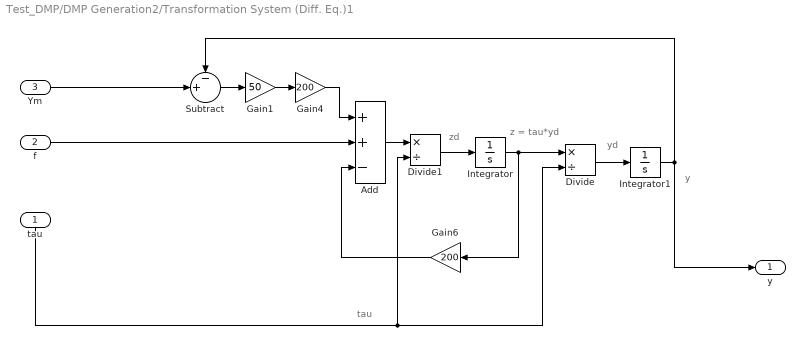
== system Test_DMP/DMP Generation2/Transformation System (Diff. Eq.)1 ==
  note: z = tau*yd
  note: yd
  note: tau
  note: zd
  note: y
  tau : Inport
  f : Inport  Port=2
  Ym : Inport  Port=3
  Add : Sum  Inputs=++-
  Divide : Product  Inputs=*/
  Divide1 : Product  Inputs=*/
  Gain1 : Gain  Gain=50
  Gain4 : Gain  Gain=200
  Gain6 : Gain  Gain=200
  Integrator : Integrator
  Integrator1 : Integrator
  Subtract : Sum  Inputs=-+|
  y : Outport
  wires:
  Ym/1 -> Subtract/2
  Gain6/1 -> Add/3
  Integrator/1 -> Divide/1, Gain6/1
  Integrator1/1 -> Subtract/1, y/1
  f/1 -> Add/2
  tau/1 -> Divide1/2, Divide/2
  Divide1/1 -> Integrator/1
  Subtract/1 -> Gain1/1
  Gain4/1 -> Add/1
  Gain1/1 -> Gain4/1
  Add/1 -> Divide1/1
  Divide/1 -> Integrator1/1

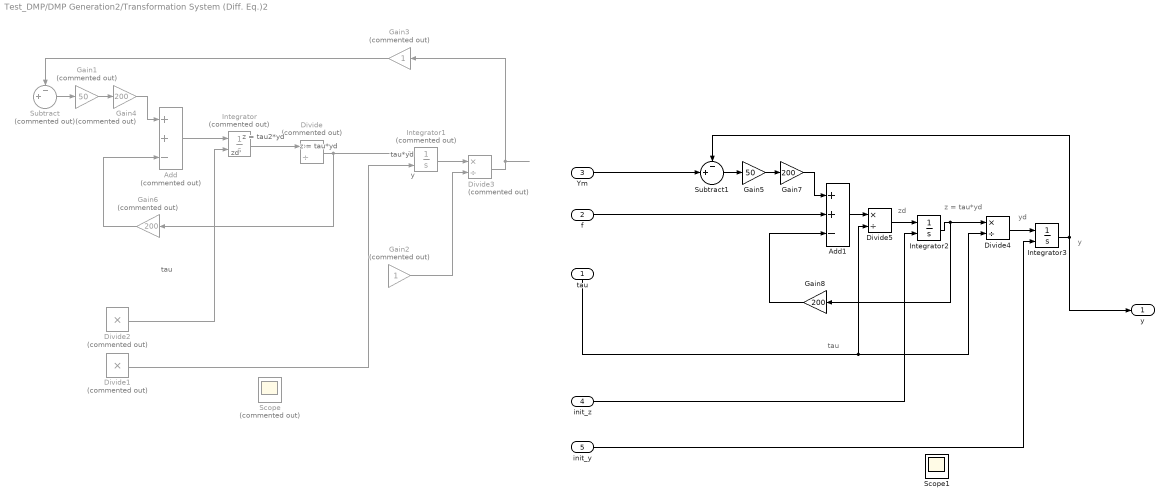
== system Test_DMP/DMP Generation2/Transformation System (Diff. Eq.)2 ==
  note: z = tau*yd
  note: yd
  note: tau
  note: zd
  note: y
  note: z = tau*yd
  note: z = tau2*yd
  note: tau*yd
  note: tau
  note: zd
  note: y
  tau : Inport
  f : Inport  Port=2
  Ym : Inport  Port=3
  init_z : Inport  Port=4
  init_y : Inport  Port=5
  Add : Sum  Commented=on  Inputs=++-
  Add1 : Sum  Inputs=++-
  Divide : Product  Commented=on  Inputs=*/
  Divide1 : Product  Commented=on  Inputs=**
  Divide2 : Product  Commented=on  Inputs=**
  Divide3 : Product  Commented=on  Inputs=*/
  Divide4 : Product  Inputs=*/
  Divide5 : Product  Inputs=*/
  Gain1 : Gain  Commented=on  Gain=50
  Gain2 : Gain  Commented=on
  Gain3 : Gain  Commented=on
  Gain4 : Gain  Commented=on  Gain=200
  Gain5 : Gain  Gain=50
  Gain6 : Gain  Commented=on  Gain=200
  Gain7 : Gain  Gain=200
  Gain8 : Gain  Gain=200
  Integrator : Integrator  Commented=on  InitialConditionSource=external  LimitOutput=on
  Integrator1 : Integrator  Commented=on  InitialConditionSource=external
  Integrator2 : Integrator  InitialConditionSource=external
  Integrator3 : Integrator  InitialConditionSource=external
  Scope : Scope  Commented=on
  Scope1 : Scope
  Subtract : Sum  Commented=on  Inputs=-+|
  Subtract1 : Sum  Inputs=-+|
  y : Outport
  wires:
  Divide4/1 -> Integrator3/1
  Add1/1 -> Divide5/1
  Gain5/1 -> Gain7/1
  Subtract1/1 -> Gain5/1
  tau/1 -> Divide5/2, Divide4/2
  Gain7/1 -> Add1/1
  Divide5/1 -> Integrator2/1
  f/1 -> Add1/2
  Integrator3/1 -> y/1, Subtract1/1
  Gain8/1 -> Add1/3
  init_z/1 -> Integrator2/2
  Integrator2/1 -> Divide4/1, Gain8/1
  Ym/1 -> Subtract1/2
  init_y/1 -> Integrator3/2
  Gain3/1 -> Subtract/1
  Gain2/1 -> Divide3/2
  Integrator1/1 -> Divide3/1
  Divide1/1 -> Integrator1/2
  Divide2/1 -> Integrator/2
  ? -> Divide1/2
  ? -> Divide2/2
  ? -> Subtract/2
  Gain6/1 -> Add/3
  Integrator/1 -> Divide/1
  Divide3/1 -> Gain3/1
  ? -> Add/2
  ? -> Divide/2, Gain2/1, Divide2/1, Divide1/1
  Add/1 -> Integrator/1
  Subtract/1 -> Gain1/1
  Gain4/1 -> Add/1
  Gain1/1 -> Gain4/1
  Divide/1 -> Integrator1/1, Gain6/1

== matlab function Test_DMP/DMP Generation/DMP+Initiation1 ==
  data: t input; init_pos input; DMP_rev output; Y input
function DMP_rev = fcn(t, init_pos, Y)

yy = 0;

for j = 1:6
    
    %% Knee Trajectories saturation
    if j==2 || j==5
        if Y(j)<0
            Y(j) = 0;
        end
    end
    
    %% Smoothening of the Hip Trajectories Notches
%     if t>156*dt && t<174*dt
%         
%         if j==1 || j==4
%             if t == 156*dt
%                 yy = Y(j);
%             end
%             
%             Y(j)=yy+(Y(j)-yy)*(t/dt-156)'/17;
%         end
%     end
    
    %% Set up the initial trajectory bridging the double-stance phase to the onset of the DMP Trajectory
    if t<=.01
        if j==1
            Y(j) = 0;
        elseif j==2
            Y(j) = 0;
        elseif j==4
            Y(j) = 0;
        elseif  j==3 || j==6
            Y(j) = 0;
        elseif j==5
            Y(j) = 0;
        end
        
    %%%    
%     elseif t<=.59
%         if j==1
%             Y(j) = -22.09*t/.59;
%         elseif j==2
%             Y(j) = 5.86*t/.59;
%         elseif j==4     % right hip in orange
%             Y(j) = -4.7*t/.59;
%         elseif  j==3 || j==6    % 6: right ankle in yellow
%             Y(j) = 0;
%         elseif j==5     % right knee in blue
%             Y(j) = -(6/.29^2)*(t-.29).^2+3;
%             if Y(j)<0
%                 Y(j)=0;
%             end
%             
% 
%         end
       %%%% 
%     elseif t>.45 && t<=.475
%         Y(4)=4.7-(t-.45)/.025*.75;
    %%%%    
    elseif t<=.67
        if j==1
            Y(j) = +23/(.39)^2*(t-.39).^2-23;
        elseif j==4
            Y(j) = 5*t/.65;
        elseif  j==3   % 6: right ankle in yellow
            Y(j) = -0*t/.65;
        elseif  j==6   % 6: right ankle in yellow
            Y(j) = 0;
        elseif j==2
            Y(j)= 14*t/.6;
            
        elseif j==5     % right knee in blue
            Y(j) = -(10/.29^2)*(t-.29).^2+10;
            if Y(j)<0
                Y(j)=0;
            end
            

        end
    %%%%%    
    end
    
    %% The final revised DMP
    DMP_rev = Y(end:-1:1);
end

== matlab function Test_DMP/DMP Generation1/DMP+Initiation1 ==
  data: t input; init_pos input; DMP_rev output; Y input
function DMP_rev = fcn(t, init_pos, Y)

yy = 0;

for j = 1:6
    
    %% Knee Trajectories saturation
    if j==2 || j==5
        if Y(j)<0
            Y(j) = 0;
        end
    end
    
    %% Smoothening of the Hip Trajectories Notches
%     if t>156*dt && t<174*dt
%         
%         if j==1 || j==4
%             if t == 156*dt
%                 yy = Y(j);
%             end
%             
%             Y(j)=yy+(Y(j)-yy)*(t/dt-156)'/17;
%         end
%     end
    
    %% Set up the initial trajectory bridging the double-stance phase to the onset of the DMP Trajectory
    if t<=.01
        if j==1
            Y(j) = 0;
        elseif j==2
            Y(j) = 0;
        elseif j==4
            Y(j) = 0;
        elseif  j==3 || j==6
            Y(j) = 0;
        elseif j==5
            Y(j) = 0;
        end
        
    %%%    
%     elseif t<=.59
%         if j==1
%             Y(j) = -22.09*t/.59;
%         elseif j==2
%             Y(j) = 5.86*t/.59;
%         elseif j==4     % right hip in orange
%             Y(j) = -4.7*t/.59;
%         elseif  j==3 || j==6    % 6: right ankle in yellow
%             Y(j) = 0;
%         elseif j==5     % right knee in blue
%             Y(j) = -(6/.29^2)*(t-.29).^2+3;
%             if Y(j)<0
%                 Y(j)=0;
%             end
%             
% 
%         end
       %%%% 
%     elseif t>.45 && t<=.475
%         Y(4)=4.7-(t-.45)/.025*.75;
    %%%%    
    elseif t<=.67
        if j==1
            Y(j) = +23/(.39)^2*(t-.39).^2-23;
        elseif j==4
            Y(j) = 5*t/.65;
        elseif  j==3   % 6: right ankle in yellow
            Y(j) = -0*t/.65;
        elseif  j==6   % 6: right ankle in yellow
            Y(j) = 0;
        elseif j==2
            Y(j)= 14*t/.6;
            
        elseif j==5     % right knee in blue
            Y(j) = -(10/.29^2)*(t-.29).^2+10;
            if Y(j)<0
                Y(j)=0;
            end
            

        end
    %%%%%    
    end
    
    %% The final revised DMP
    DMP_rev = Y(end:-1:1);
end

== matlab function Test_DMP/DMP Generation1/DMP+Initiation2 ==
  data: t input; dt input; DMP_rev output; Y input
function DMP_rev = fcn(t, dt, Y)

yy = 0;

for j = 1:6
    
    %% Knee Trajectories saturation
    if j==2 || j==5
        if Y(j)<0
            Y(j) = 0;
        end
    end
    
    %% Smoothening of the Hip Trajectories Notches
%     if t>156*dt && t<174*dt
%         
%         if j==1 || j==4
%             if t == 156*dt
%                 yy = Y(j);
%             end
%             
%             Y(j)=yy+(Y(j)-yy)*(t/dt-156)'/17;
%         end
%     end
    
    %% Set up the initial trajectory bridging the double-stance phase to the onset of the DMP Trajectory
    if t<=.01
        if j==1
            Y(j) = 0;
        elseif j==2
            Y(j) = 0;
        elseif j==4
            Y(j) = 0;
        elseif  j==3 || j==6
            Y(j) = 0;
        elseif j==5
            Y(j) = 0;
        end
    elseif t<=.45
        if j==1
            Y(j) = -22.09*t/.45;
        elseif j==2
            Y(j) = 5.86*t/.45;
        elseif j==4     % right hip in orange
            Y(j) = 4.7*t/.45;
        elseif  j==3 || j==6    % 6: right ankle in yellow
            Y(j) = 0;
        elseif j==5     % right knee in blue
            Y(j) = -(6/.2^2)*(t-.2).^2+3;
            if Y(j)<0
                Y(j)=0;
            end

        end
        
    elseif t>.45 && t<=.475
        Y(4)=4.7-(t-.45)/.025*.75;
        
    
        
    end
    
    %% The final revised DMP
    DMP_rev = Y(end:-1:1);
end

== matlab function Test_DMP/DMP Generation1/DMP+Initiation3 ==
  data: t input; dt input; DMP_rev output; Y input
function DMP_rev = fcn(t, dt, Y)

yy = 0;

for j = 1:6
    
    %% Knee Trajectories saturation
    if j==2 || j==5
        if Y(j)<0
            Y(j) = 0;
        end
    end
    
    %% Smoothening of the Hip Trajectories Notches
%     if t>156*dt && t<174*dt
%         
%         if j==1 || j==4
%             if t == 156*dt
%                 yy = Y(j);
%             end
%             
%             Y(j)=yy+(Y(j)-yy)*(t/dt-156)'/17;
%         end
%     end
    
    %% Set up the initial trajectory bridging the double-stance phase to the onset of the DMP Trajectory
    
    if t<=.0001
        if j==1
            Y(j) = 0;
        elseif j==2
            Y(j) = 0;
        elseif j==4
            Y(j) = 0;
        elseif  j==3 || j==6
            Y(j) = 0;
        elseif j==5
            Y(j) = 0;
        end
        
    elseif t<.59
        if j==1
            Y(j) = -22.09*t/.59;
        elseif j==2
            Y(j) = 5.86*t/.59;
        elseif j==4
            Y(j) = 8.66*t/.59;
        elseif  j==3 || j==6
            Y(j) = 0;
        elseif j==5
            Y(j) = -(6/.29^2)*(t-.29).^2+3;
        end
               
    end
    
    %% The final revised DMP
    DMP_rev = Y(end:-1:1);
end

== matlab function Test_DMP/DMP Generation/Forcing_Term1 ==
  data: f output; PSI input; W input; Amp input
function f = fcn(PSI,W,Amp)

f = zeros(1,6);

for i=1:6
%     amp = Amp(i);
    w   = W(:,i);
    psi = PSI(:,i);
    
    f(i)            = sum(w.*psi)/sum(psi+1.e-10) * Amp;
    
end
end

== matlab function Test_DMP/DMP Generation/Gaussian_fun1 ==
  data: PSI output; Phi input
function PSI = fcn(Phi)

n_rfs  = 50;    % number of kernel functions

% the time constants for chosen for critical damping

c       = 2*pi*(1/n_rfs:1/n_rfs:1)';
D       = ones(n_rfs,1)*.1*n_rfs^2;

PSI = zeros(n_rfs,6);

for i=1:6
    
    p = Phi;
    
    PSI(:,i) = exp(D.*(cos(p-c)-1));
    
end

== matlab function Test_DMP/DMP Generation1/DMP+Initiation4 ==
  data: t input; init_pos input; DMP_rev output; Y input
function DMP_rev = fcn(t, init_pos, Y)

yy = 0;

for j = 1:6
    
    %% Knee Trajectories saturation
    if j==2 || j==5
        if Y(j)<0
            Y(j) = 0;
        end
    end
    
    %% Smoothening of the Hip Trajectories Notches
%     if t>156*dt && t<174*dt
%         
%         if j==1 || j==4
%             if t == 156*dt
%                 yy = Y(j);
%             end
%             
%             Y(j)=yy+(Y(j)-yy)*(t/dt-156)'/17;
%         end
%     end
    
    %% Set up the initial trajectory bridging the double-stance phase to the onset of the DMP Trajectory
%     if t<=.01
%         if j==1
%             Y(j) = 0;
%         elseif j==2
%             Y(j) = 0;
%         elseif j==4
%             Y(j) = 0;
%         elseif  j==3 || j==6
%             Y(j) = 0;
%         elseif j==5
%             Y(j) = 0;
%         end
%         
%     %%%    
% %     elseif t<=.59
% %         if j==1
% %             Y(j) = -22.09*t/.59;
% %         elseif j==2
% %             Y(j) = 5.86*t/.59;
% %         elseif j==4     % right hip in orange
% %             Y(j) = -4.7*t/.59;
% %         elseif  j==3 || j==6    % 6: right ankle in yellow
% %             Y(j) = 0;
% %         elseif j==5     % right knee in blue
% %             Y(j) = -(6/.29^2)*(t-.29).^2+3;
% %             if Y(j)<0
% %                 Y(j)=0;
% %             end
% %             
% % 
% %         end
%        %%%% 
% %     elseif t>.45 && t<=.475
% %         Y(4)=4.7-(t-.45)/.025*.75;
%     %%%%    
%     elseif t<=.67
%         if j==1
%             Y(j) = +23/(.39)^2*(t-.39).^2-23;
%         elseif j==4
%             Y(j) = 5*t/.65;
%         elseif  j==3   % 6: right ankle in yellow
%             Y(j) = -0*t/.65;
%         elseif  j==6   % 6: right ankle in yellow
%             Y(j) = 0;
%         elseif j==2
%             Y(j)= 14*t/.6;
%             
%         elseif j==5     % right knee in blue
%             Y(j) = -(10/.29^2)*(t-.29).^2+10;
%             if Y(j)<0
%                 Y(j)=0;
%             end
%             
% 
%         end
%     %%%%%    
%     end
    
    %% The final revised DMP
    DMP_rev = Y(end:-1:1);
end

== matlab function Test_DMP/DMP Generation1/Forcing_Term1 ==
  data: f output; PSI input; W input; Amp input
function f = fcn(PSI,W,Amp)

f = zeros(1,6);

for i=1:6
%     amp = Amp(i);
    w   = W(:,i);
    psi = PSI(:,i);
    
    f(i)            = sum(w.*psi)/sum(psi+1.e-10) * Amp;
    
end
end

== matlab function Test_DMP/DMP Generation1/Forcing_Term2 ==
  data: f output; PSI input; W input; Amp input
function f = fcn(PSI,W,Amp)

f = zeros(1,6);

for i=1:6
%     amp = Amp(i);
    w   = W(:,i);
    psi = PSI(:,i);
    A = Amp(i);
    
    f(i)            = sum(w.*psi)/sum(psi+1.e-10) * A;
    
end
end

== matlab function Test_DMP/DMP Generation/DMP+Initiation2 ==
  data: t input; dt input; DMP_rev output; Y input
function DMP_rev = fcn(t, dt, Y)

yy = 0;

for j = 1:6
    
    %% Knee Trajectories saturation
    if j==2 || j==5
        if Y(j)<0
            Y(j) = 0;
        end
    end
    
    %% Smoothening of the Hip Trajectories Notches
%     if t>156*dt && t<174*dt
%         
%         if j==1 || j==4
%             if t == 156*dt
%                 yy = Y(j);
%             end
%             
%             Y(j)=yy+(Y(j)-yy)*(t/dt-156)'/17;
%         end
%     end
    
    %% Set up the initial trajectory bridging the double-stance phase to the onset of the DMP Trajectory
    if t<=.01
        if j==1
            Y(j) = 0;
        elseif j==2
            Y(j) = 0;
        elseif j==4
            Y(j) = 0;
        elseif  j==3 || j==6
            Y(j) = 0;
        elseif j==5
            Y(j) = 0;
        end
    elseif t<=.45
        if j==1
            Y(j) = -22.09*t/.45;
        elseif j==2
            Y(j) = 5.86*t/.45;
        elseif j==4     % right hip in orange
            Y(j) = 4.7*t/.45;
        elseif  j==3 || j==6    % 6: right ankle in yellow
            Y(j) = 0;
        elseif j==5     % right knee in blue
            Y(j) = -(6/.2^2)*(t-.2).^2+3;
            if Y(j)<0
                Y(j)=0;
            end

        end
        
    elseif t>.45 && t<=.475
        Y(4)=4.7-(t-.45)/.025*.75;
        
    
        
    end
    
    %% The final revised DMP
    DMP_rev = Y(end:-1:1);
end

== matlab function Test_DMP/DMP Generation/DMP+Initiation3 ==
  data: t input; dt input; DMP_rev output; Y input
function DMP_rev = fcn(t, dt, Y)

yy = 0;

for j = 1:6
    
    %% Knee Trajectories saturation
    if j==2 || j==5
        if Y(j)<0
            Y(j) = 0;
        end
    end
    
    %% Smoothening of the Hip Trajectories Notches
%     if t>156*dt && t<174*dt
%         
%         if j==1 || j==4
%             if t == 156*dt
%                 yy = Y(j);
%             end
%             
%             Y(j)=yy+(Y(j)-yy)*(t/dt-156)'/17;
%         end
%     end
    
    %% Set up the initial trajectory bridging the double-stance phase to the onset of the DMP Trajectory
    
    if t<=.0001
        if j==1
            Y(j) = 0;
        elseif j==2
            Y(j) = 0;
        elseif j==4
            Y(j) = 0;
        elseif  j==3 || j==6
            Y(j) = 0;
        elseif j==5
            Y(j) = 0;
        end
        
    elseif t<.59
        if j==1
            Y(j) = -22.09*t/.59;
        elseif j==2
            Y(j) = 5.86*t/.59;
        elseif j==4
            Y(j) = 8.66*t/.59;
        elseif  j==3 || j==6
            Y(j) = 0;
        elseif j==5
            Y(j) = -(6/.29^2)*(t-.29).^2+3;
        end
               
    end
    
    %% The final revised DMP
    DMP_rev = Y(end:-1:1);
end

== matlab function Test_DMP/DMP Generation/Forcing_Term2 ==
  data: f output; PSI input; W input; Amp input
function f = fcn(PSI,W,Amp)

f = zeros(1,6);

for i=1:6
%     amp = Amp(i);
    w   = W(:,i);
    psi = PSI(:,i);
    A = Amp(i);
    
    f(i)            = sum(w.*psi)/sum(psi+1.e-10) * A;
    
end
end

== matlab function Test_DMP/DMP Generation/Gaussian_fun2 ==
  data: PSI output; Phi input
function PSI = fcn(Phi)

n_rfs  = 100;    % number of kernel functions

% the time constants for chosen for critical damping

c       = 2*pi*(1/n_rfs:1/n_rfs:1)';
D       = ones(n_rfs,1)*.1*n_rfs^2;

PSI = zeros(n_rfs,6);

for i=1:6
    
    p = Phi;
    
    PSI(:,i) = exp(D.*(cos(p-c)-1));
    
end

== matlab function Test_DMP/DMP Generation/Initial States ==
  data: tau input; pos_i output; init_pos input; init_vel input; z_i output
function [pos_i, z_i] = fcn(tau,init_pos,init_vel)

pos_i = zeros(6,1);
z_i   = zeros(6,1);
for i=1:6

    pos_i(i,1)   = init_pos(i,1);
    vel_i   = init_vel(i,1);
    z_i(i,1)     = vel_i*tau;
        
end
    
end

== matlab function Test_DMP/DMP Generation/DMP+Initiation4 ==
  data: t input; init_pos input; DMP_rev output; Y input
function DMP_rev = fcn(t, init_pos, Y)

yy = 0;

for j = 1:6
    
    %% Knee Trajectories saturation
    if j==2 || j==5
        if Y(j)<0
            Y(j) = 0;
        end
    end
    
    %% Smoothening of the Hip Trajectories Notches
%     if t>156*dt && t<174*dt
%         
%         if j==1 || j==4
%             if t == 156*dt
%                 yy = Y(j);
%             end
%             
%             Y(j)=yy+(Y(j)-yy)*(t/dt-156)'/17;
%         end
%     end
    
    %% Set up the initial trajectory bridging the double-stance phase to the onset of the DMP Trajectory
%     if t<=.01
%         if j==1
%             Y(j) = 0;
%         elseif j==2
%             Y(j) = 0;
%         elseif j==4
%             Y(j) = 0;
%         elseif  j==3 || j==6
%             Y(j) = 0;
%         elseif j==5
%             Y(j) = 0;
%         end
%         
%     %%%    
% %     elseif t<=.59
% %         if j==1
% %             Y(j) = -22.09*t/.59;
% %         elseif j==2
% %             Y(j) = 5.86*t/.59;
% %         elseif j==4     % right hip in orange
% %             Y(j) = -4.7*t/.59;
% %         elseif  j==3 || j==6    % 6: right ankle in yellow
% %             Y(j) = 0;
% %         elseif j==5     % right knee in blue
% %             Y(j) = -(6/.29^2)*(t-.29).^2+3;
% %             if Y(j)<0
% %                 Y(j)=0;
% %             end
% %             
% % 
% %         end
%        %%%% 
% %     elseif t>.45 && t<=.475
% %         Y(4)=4.7-(t-.45)/.025*.75;
%     %%%%    
%     elseif t<=.67
%         if j==1
%             Y(j) = +23/(.39)^2*(t-.39).^2-23;
%         elseif j==4
%             Y(j) = 5*t/.65;
%         elseif  j==3   % 6: right ankle in yellow
%             Y(j) = -0*t/.65;
%         elseif  j==6   % 6: right ankle in yellow
%             Y(j) = 0;
%         elseif j==2
%             Y(j)= 14*t/.6;
%             
%         elseif j==5     % right knee in blue
%             Y(j) = -(10/.29^2)*(t-.29).^2+10;
%             if Y(j)<0
%                 Y(j)=0;
%             end
%             
% 
%         end
%     %%%%%    
%     end
    
    %% The final revised DMP
    DMP_rev = Y(end:-1:1);
end

== matlab function Test_DMP/DMP Generation1/Gaussian_fun1 ==
  data: PSI output; Phi input
function PSI = fcn(Phi)

n_rfs  = 50;    % number of kernel functions

% the time constants for chosen for critical damping

c       = 2*pi*(1/n_rfs:1/n_rfs:1)';
D       = ones(n_rfs,1)*.1*n_rfs^2;

PSI = zeros(n_rfs,6);

for i=1:6
    
    p = Phi;
    
    PSI(:,i) = exp(D.*(cos(p-c)-1));
    
end

== matlab function Test_DMP/DMP Generation1/Gaussian_fun2 ==
  data: PSI output; Phi input
function PSI = fcn(Phi)

n_rfs  = 100;    % number of kernel functions

% the time constants for chosen for critical damping

c       = 2*pi*(1/n_rfs:1/n_rfs:1)';
D       = ones(n_rfs,1)*.1*n_rfs^2;

PSI = zeros(n_rfs,6);

for i=1:6
    
    p = Phi;
    
    PSI(:,i) = exp(D.*(cos(p-c)-1));
    
end

== matlab function Test_DMP/DMP Generation1/Initial States ==
  data: tau input; pos_i output; init_pos input; init_vel input; z_i output
function [pos_i, z_i] = fcn(tau,init_pos,init_vel)

pos_i = zeros(6,1);
z_i   = zeros(6,1);
for i=1:6

    pos_i(i,1)   = init_pos(i,1);
    vel_i   = init_vel(i,1);
    z_i(i,1)     = vel_i*tau;
        
end
    
end

== matlab function Test_DMP/DMP Generation2/DMP+Initiation1 ==
  data: t input; init_pos input; DMP_rev output; Y input
function DMP_rev = fcn(t, init_pos, Y)

yy = 0;

for j = 1:6
    
    %% Knee Trajectories saturation
    if j==2 || j==5
        if Y(j)<0
            Y(j) = 0;
        end
    end
    
    %% Smoothening of the Hip Trajectories Notches
%     if t>156*dt && t<174*dt
%         
%         if j==1 || j==4
%             if t == 156*dt
%                 yy = Y(j);
%             end
%             
%             Y(j)=yy+(Y(j)-yy)*(t/dt-156)'/17;
%         end
%     end
    
    %% Set up the initial trajectory bridging the double-stance phase to the onset of the DMP Trajectory
    if t<=.01
        if j==1
            Y(j) = 0;
        elseif j==2
            Y(j) = 0;
        elseif j==4
            Y(j) = 0;
        elseif  j==3 || j==6
            Y(j) = 0;
        elseif j==5
            Y(j) = 0;
        end
        
    %%%    
%     elseif t<=.59
%         if j==1
%             Y(j) = -22.09*t/.59;
%         elseif j==2
%             Y(j) = 5.86*t/.59;
%         elseif j==4     % right hip in orange
%             Y(j) = -4.7*t/.59;
%         elseif  j==3 || j==6    % 6: right ankle in yellow
%             Y(j) = 0;
%         elseif j==5     % right knee in blue
%             Y(j) = -(6/.29^2)*(t-.29).^2+3;
%             if Y(j)<0
%                 Y(j)=0;
%             end
%             
% 
%         end
       %%%% 
%     elseif t>.45 && t<=.475
%         Y(4)=4.7-(t-.45)/.025*.75;
    %%%%    
    elseif t<=.67
        if j==1
            Y(j) = +23/(.39)^2*(t-.39).^2-23;
        elseif j==4
            Y(j) = 5*t/.65;
        elseif  j==3   % 6: right ankle in yellow
            Y(j) = -0*t/.65;
        elseif  j==6   % 6: right ankle in yellow
            Y(j) = 0;
        elseif j==2
            Y(j)= 14*t/.6;
            
        elseif j==5     % right knee in blue
            Y(j) = -(10/.29^2)*(t-.29).^2+10;
            if Y(j)<0
                Y(j)=0;
            end
            

        end
    %%%%%    
    end
    
    %% The final revised DMP
    DMP_rev = Y(end:-1:1);
end
